simulink subsystem "rss_MotoSpdLoLvl1Dia"  (R2023a)
settings: Solver=VariableStepAuto  StartTime=0.0  StopTime=10.0  RelTol=1e-3
undefined symbols (not defined in the file): Cdbl_nElecAgSpdMaxVal, ENM_MOTO_STATUS, ENM_TYPE_FALT, Gs16_nMaxMotoSpdDvtConfTrs_C, Gs16_nMinMotoSpdDvtRcvyTrs_C, Gu16_ctMaxMotoSpdDvtConfCnt_C, Gu16_ctMinMotoSpdDvtRcvyCnt_C
libraries: simulink x2, lib_conversion x1, vhit_control_library x1, lib_fault_definiteness x1
settings Model: DefaultTestHarness=rss_DeratingFlag_thu  Creator=YXQ1WX  LastModifiedBy=xiaoqiang.yuan
settings OptimizationCC: ReuseModelBlockBuffer=off

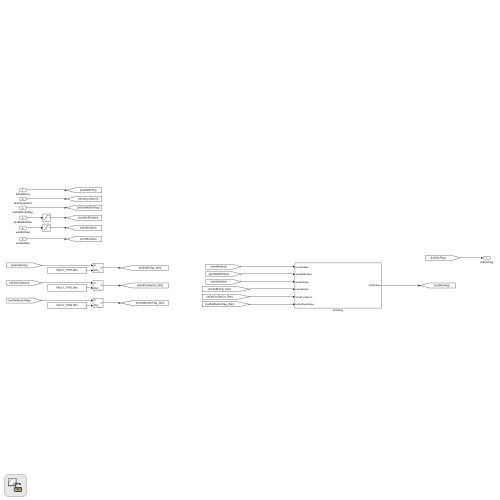
[thumbnail: Simulink's stored preview of the top-level diagram]
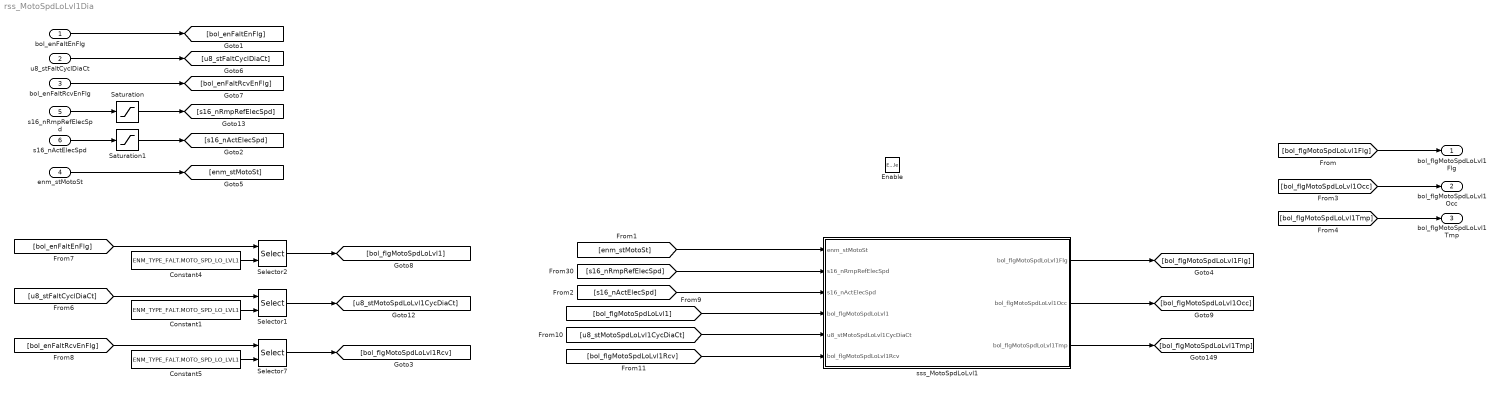
== system rss_MotoSpdLoLvl1Dia ==
  bol_enFaltEnFlg : Inport  OutDataTypeStr=boolean
  u8_stFaltCyclDiaCt : Inport  Port=2  OutDataTypeStr=uint8
  bol_enFaltRcvEnFlg : Inport  Port=3  OutDataTypeStr=boolean
  enm_stMotoSt : Inport  Port=4  OutDataTypeStr=Enum: ENM_MOTO_STATUS
  s16_nRmpRefElecSpd : Inport  Port=5  OutDataTypeStr=dt_Standardize_s16p15b0
  s16_nActElecSpd : Inport  Port=6  OutDataTypeStr=dt_Standardize_s16p15b0
  Enable : EnablePort
  Constant1 : Constant  Value=ENM_TYPE_FALT.MOTO_SPD_LO_LVL1
  Constant4 : Constant  Value=ENM_TYPE_FALT.MOTO_SPD_LO_LVL1
  Constant5 : Constant  Value=ENM_TYPE_FALT.MOTO_SPD_LO_LVL1
  Saturation : Saturate  UpperLimit=Cdbl_nElecAgSpdMaxVal  LowerLimit=-Cdbl_nElecAgSpdMaxVal
  Saturation1 : Saturate  UpperLimit=Cdbl_nElecAgSpdMaxVal  LowerLimit=-Cdbl_nElecAgSpdMaxVal
  Selector1 : Selector  IndexMode=Zero-based  InputPortWidth=Cdbl_numFaltDiaNum  IndexOptions=Index vector (port)  Indices=[1 3]  OutputSizes=1
  Selector2 : Selector  IndexMode=Zero-based  InputPortWidth=Cdbl_numFaltDiaNum  IndexOptions=Index vector (port)  Indices=[1 3]  OutputSizes=1
  Selector7 : Selector  IndexMode=Zero-based  InputPortWidth=Cdbl_numFaltDiaNum  IndexOptions=Index vector (port)  Indices=[1 3]  OutputSizes=1
  sss_MotoSpdLoLvl1 : Subsystem
  bol_flgMotoSpdLoLvl1Flg : Outport  OutDataTypeStr=boolean
  bol_flgMotoSpdLoLvl1Occ : Outport  Port=2  OutDataTypeStr=boolean
  bol_flgMotoSpdLoLvl1Tmp : Outport  Port=3  OutDataTypeStr=boolean
  wires:
  [bol_flgMotoSpdLoLvl1Flg] -> bol_flgMotoSpdLoLvl1Flg/1
  enm_stMotoSt/1 -> [enm_stMotoSt]
  s16_nRmpRefElecSpd/1 -> Saturation/1
  s16_nActElecSpd/1 -> Saturation1/1
  Saturation/1 -> [s16_nRmpRefElecSpd]
  Saturation1/1 -> [s16_nActElecSpd]
  bol_enFaltEnFlg/1 -> [bol_enFaltEnFlg]
  bol_enFaltRcvEnFlg/1 -> [bol_enFaltRcvEnFlg]
  u8_stFaltCyclDiaCt/1 -> [u8_stFaltCyclDiaCt]
  Selector2/1 -> [bol_flgMotoSpdLoLvl1]
  Constant5/1 -> Selector7/2
  Constant1/1 -> Selector1/2
  Selector1/1 -> [u8_stMotoSpdLoLvl1CycDiaCt]
  [u8_stFaltCyclDiaCt] -> Selector1/1
  [bol_enFaltEnFlg] -> Selector2/1
  [bol_enFaltRcvEnFlg] -> Selector7/1
  Selector7/1 -> [bol_flgMotoSpdLoLvl1Rcv]
  Constant4/1 -> Selector2/2
  [enm_stMotoSt] -> sss_MotoSpdLoLvl1/1(enm_stMotoSt)
  [s16_nRmpRefElecSpd] -> sss_MotoSpdLoLvl1/2(s16_nRmpRefElecSpd)
  [s16_nActElecSpd] -> sss_MotoSpdLoLvl1/3(s16_nActElecSpd)
  sss_MotoSpdLoLvl1/1(bol_flgMotoSpdLoLvl1Flg) -> [bol_flgMotoSpdLoLvl1Flg]
  [bol_flgMotoSpdLoLvl1] -> sss_MotoSpdLoLvl1/4(bol_flgMotoSpdLoLvl1)
  [u8_stMotoSpdLoLvl1CycDiaCt] -> sss_MotoSpdLoLvl1/5(u8_stMotoSpdLoLvl1CycDiaCt)
  [bol_flgMotoSpdLoLvl1Rcv] -> sss_MotoSpdLoLvl1/6(bol_flgMotoSpdLoLvl1Rcv)
  sss_MotoSpdLoLvl1/2(bol_flgMotoSpdLoLvl1Occ) -> [bol_flgMotoSpdLoLvl1Occ]
  [bol_flgMotoSpdLoLvl1Occ] -> bol_flgMotoSpdLoLvl1Occ/1
  [bol_flgMotoSpdLoLvl1Tmp] -> bol_flgMotoSpdLoLvl1Tmp/1
  sss_MotoSpdLoLvl1/3(bol_flgMotoSpdLoLvl1Tmp) -> [bol_flgMotoSpdLoLvl1Tmp]

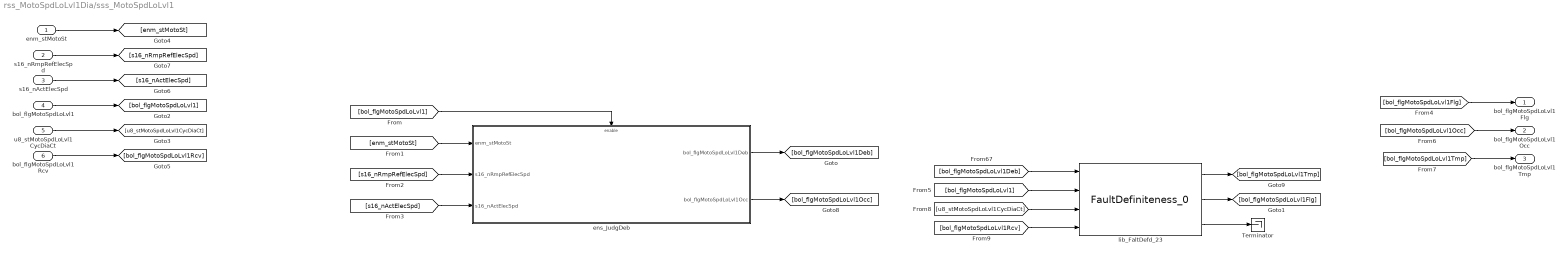
== system rss_MotoSpdLoLvl1Dia/sss_MotoSpdLoLvl1 ==
  enm_stMotoSt : Inport
  s16_nRmpRefElecSpd : Inport  Port=2
  s16_nActElecSpd : Inport  Port=3
  bol_flgMotoSpdLoLvl1 : Inport  Port=4
  u8_stMotoSpdLoLvl1CycDiaCt : Inport  Port=5
  bol_flgMotoSpdLoLvl1Rcv : Inport  Port=6
  Terminator : Terminator
  ens_JudgDeb : Subsystem
  lib_FaltDefd_23 : lib_fault_definiteness/FaultDefiniteness_0  lb_FaltWaitRecvCnt=Gu16_ctMaxMotoSpdDvtConfCnt_C
  bol_flgMotoSpdLoLvl1Flg : Outport
  bol_flgMotoSpdLoLvl1Occ : Outport  Port=2
  bol_flgMotoSpdLoLvl1Tmp : Outport  Port=3
  wires:
  [bol_flgMotoSpdLoLvl1Tmp] -> bol_flgMotoSpdLoLvl1Tmp/1
  [bol_flgMotoSpdLoLvl1Occ] -> bol_flgMotoSpdLoLvl1Occ/1
  ens_JudgDeb/2(bol_flgMotoSpdLoLvl1Occ) -> [bol_flgMotoSpdLoLvl1Occ]
  lib_FaltDefd_23/1 -> [bol_flgMotoSpdLoLvl1Tmp]
  lib_FaltDefd_23/2 -> [bol_flgMotoSpdLoLvl1Flg]
  lib_FaltDefd_23/3 -> Terminator/1
  [bol_flgMotoSpdLoLvl1Flg] -> bol_flgMotoSpdLoLvl1Flg/1
  ens_JudgDeb/1(bol_flgMotoSpdLoLvl1Deb) -> [bol_flgMotoSpdLoLvl1Deb]
  [bol_flgMotoSpdLoLvl1Deb] -> lib_FaltDefd_23/1
  [bol_flgMotoSpdLoLvl1] -> lib_FaltDefd_23/2
  [bol_flgMotoSpdLoLvl1Rcv] -> lib_FaltDefd_23/4
  [u8_stMotoSpdLoLvl1CycDiaCt] -> lib_FaltDefd_23/3
  [s16_nActElecSpd] -> ens_JudgDeb/3(s16_nActElecSpd)
  [s16_nRmpRefElecSpd] -> ens_JudgDeb/2(s16_nRmpRefElecSpd)
  [enm_stMotoSt] -> ens_JudgDeb/1(enm_stMotoSt)
  [bol_flgMotoSpdLoLvl1] -> ens_JudgDeb/Enable
  s16_nRmpRefElecSpd/1 -> [s16_nRmpRefElecSpd]
  enm_stMotoSt/1 -> [enm_stMotoSt]
  bol_flgMotoSpdLoLvl1Rcv/1 -> [bol_flgMotoSpdLoLvl1Rcv]
  s16_nActElecSpd/1 -> [s16_nActElecSpd]
  bol_flgMotoSpdLoLvl1/1 -> [bol_flgMotoSpdLoLvl1]
  u8_stMotoSpdLoLvl1CycDiaCt/1 -> [u8_stMotoSpdLoLvl1CycDiaCt]

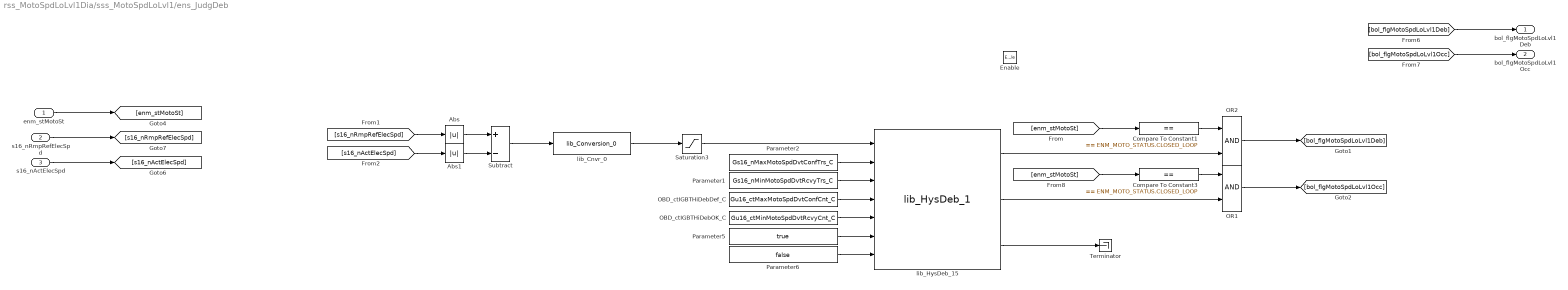
== system rss_MotoSpdLoLvl1Dia/sss_MotoSpdLoLvl1/ens_JudgDeb ==
  enm_stMotoSt : Inport
  s16_nRmpRefElecSpd : Inport  Port=2
  s16_nActElecSpd : Inport  Port=3
  Enable : EnablePort
  Abs : Abs  SaturateOnIntegerOverflow=off
  Abs1 : Abs  SaturateOnIntegerOverflow=off
  Compare To Constant1 : simulink/Logic and Bit Operations/Compare To Constant  relop===  const=ENM_MOTO_STATUS.CLOSED_LOOP  OutDataTypeStr=boolean
  Compare To Constant3 : simulink/Logic and Bit Operations/Compare To Constant  relop===  const=ENM_MOTO_STATUS.CLOSED_LOOP  OutDataTypeStr=boolean
  OBD_ctIGBTHiDebDef_C : Constant  Value=Gu16_ctMaxMotoSpdDvtConfCnt_C
  OBD_ctIGBTHiDebOK_C : Constant  Value=Gu16_ctMinMotoSpdDvtRcvyCnt_C
  OR1 : Logic  AllPortsSameDT=off  OutDataTypeStr=boolean
  OR2 : Logic  AllPortsSameDT=off  OutDataTypeStr=boolean
  Parameter1 : Constant  Value=Gs16_nMinMotoSpdDvtRcvyTrs_C  SampleTime=-1
  Parameter2 : Constant  Value=Gs16_nMaxMotoSpdDvtConfTrs_C  SampleTime=-1
  Parameter5 : Constant  Value=true  SampleTime=-1
  Parameter6 : Constant  Value=false  SampleTime=-1
  Saturation3 : Saturate  UpperLimit=Cdbl_nElecAgSpdMaxVal  LowerLimit=-Cdbl_nElecAgSpdMaxVal  OutDataTypeStr=Inherit: Inherit via back propagation
  Subtract : Sum  Inputs=+-  OutDataTypeStr=Inherit: Inherit via back propagation
  Terminator : Terminator
  lib_Cnvr_0 : lib_conversion/lib_Conversion_0  lb_parDataType=fixdt(1,16)  lb_parOutpMaxVal=2*Cdbl_nElecAgSpdMaxVal  lb_parOutpMinVal=-2*Cdbl_nElecAgSpdMaxVal  lb_parSatFlag=off
  lib_HysDeb_15 : vhit_control_library/lib_HysDeb_1  lb_parInitOutp=0
  bol_flgMotoSpdLoLvl1Deb : Outport
  bol_flgMotoSpdLoLvl1Occ : Outport  Port=2
  wires:
  OR1/1 -> [bol_flgMotoSpdLoLvl1Occ]
  lib_HysDeb_15/2 -> OR1/2
  [enm_stMotoSt] -> Compare To Constant3/1
  Compare To Constant3/1 -> OR1/1
  OR2/1 -> [bol_flgMotoSpdLoLvl1Deb]
  lib_HysDeb_15/1 -> OR2/2
  [bol_flgMotoSpdLoLvl1Occ] -> bol_flgMotoSpdLoLvl1Occ/1
  [bol_flgMotoSpdLoLvl1Deb] -> bol_flgMotoSpdLoLvl1Deb/1
  lib_HysDeb_15/3 -> Terminator/1
  Abs1/1 -> Subtract/2
  Abs/1 -> Subtract/1
  lib_Cnvr_0/1 -> Saturation3/1
  OBD_ctIGBTHiDebOK_C/1 -> lib_HysDeb_15/5
  OBD_ctIGBTHiDebDef_C/1 -> lib_HysDeb_15/4
  Saturation3/1 -> lib_HysDeb_15/1
  Parameter6/1 -> lib_HysDeb_15/7
  Parameter5/1 -> lib_HysDeb_15/6
  Parameter1/1 -> lib_HysDeb_15/3
  Parameter2/1 -> lib_HysDeb_15/2
  enm_stMotoSt/1 -> [enm_stMotoSt]
  s16_nRmpRefElecSpd/1 -> [s16_nRmpRefElecSpd]
  s16_nActElecSpd/1 -> [s16_nActElecSpd]
  Subtract/1 -> lib_Cnvr_0/1
  Compare To Constant1/1 -> OR2/1
  [s16_nRmpRefElecSpd] -> Abs/1
  [enm_stMotoSt] -> Compare To Constant1/1
  [s16_nActElecSpd] -> Abs1/1
